simulink model "dc_1"  (Simulink 7.0)
settings: Solver=ode45  StartTime=0.0  StopTime=10.0  MaxStep=1/(2*Fc)  RelTol=1e-3
PreLoadFcn:
  | Fc    =  890e6;
  | Fsym=  20e6;
  | Frame=128;
  | D=8;
  | RRC_Delay;
undefined symbols (not defined in the file): RRC_Delay
libraries: dspbuff3 x4, dsparch4 x4, commfilt2 x2, commsink2 x1, dspstat3 x1, commdigbbndpm3 x1, commrandsrc2 x1
settings Model: Creator=dbenson  LastModifiedBy=dbenson

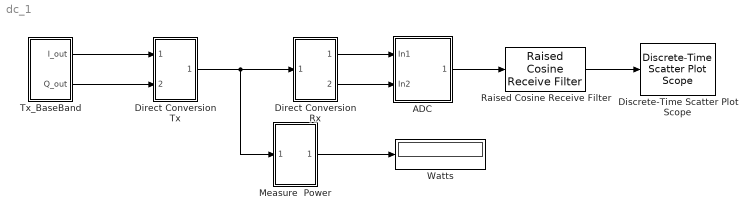
== system dc_1 ==
  ADC : Subsystem
  Direct Conversion Rx : Subsystem
  Direct Conversion Tx : Subsystem
  Discrete-Time Scatter Plot Scope : commsink2/Discrete-Time Scatter Plot Scope  Tag=ScatterPlot  SystemSampleTime=-1  sampPerSymb=1  offsetEye=0  numTraces=40  numNewFrames=10  LineMarkers=.  LineColors=b  fading=on  render=on  AxisGrid=on  xMin=-2.5  xMax=2.5  yMin=-2.5  yMax=2.5  inphaseLabel=In-phase Amplitude  quadratureLabel=Quadrature Amplitude  openScopeAtSimStart=on  FrameNumber=off  FigPos=[786 40 229 225]  figTitle=Scatter Plot  numLinesMax=8  block_type_=scatter
  Measure  Power : Subsystem
  Raised Cosine Receive Filter : commfilt2/Raised Cosine Receive Filter  DialogController=dspDDGCreate  DialogControllerArgs=DataTag1  SystemSampleTime=-1  filtType=Square root  N=8  D=RRC_Delay  R=0.25  sampMode=Frame-based  rateMode=Downsampling  downFactor=D  downOffset=6  checkGain=Normalized  filterGain=1  checkCoeff=off  variableName=rcRxFilt  launchFVT=off  roundingMode=Floor  overflowMode=off
  Tx_BaseBand : Subsystem
  Watts : Display
  wires:
  ADC/1(I/Q out) -> Raised Cosine Receive Filter/1
  Raised Cosine Receive Filter/1 -> Discrete-Time Scatter Plot Scope/1
  Tx_BaseBand/1(I_out) -> Direct Conversion Tx/1(In1)
  Tx_BaseBand/2(Q_out) -> Direct Conversion Tx/2(In2)
  Direct Conversion Rx/1(Out1) -> ADC/1(In1)
  Direct Conversion Rx/2(Out2) -> ADC/2(In2)
  Direct Conversion Tx/1(Out1) -> Direct Conversion Rx/1(In1), Measure  Power/1(In1)
  Measure  Power/1(Out1) -> Watts/1

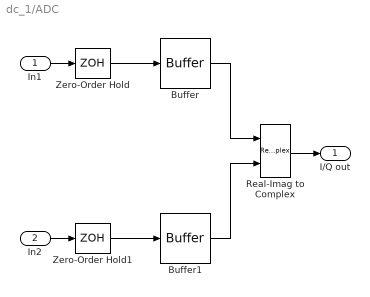
== system dc_1/ADC ==
  In1 : Inport
  In2 : Inport  Port=2
  Buffer : dspbuff3/Buffer  N=Frame  V=0  ic=0
  Buffer1 : dspbuff3/Buffer  N=Frame  V=0  ic=0
  Real-Imag to Complex : RealImagToComplex
  Zero-Order Hold : ZeroOrderHold  SampleTime=1/(D*Fsym)
  Zero-Order Hold1 : ZeroOrderHold  SampleTime=1/(D*Fsym)
  I/Q out : Outport
  wires:
  In1/1 -> Zero-Order Hold/1
  Zero-Order Hold/1 -> Buffer/1
  In2/1 -> Zero-Order Hold1/1
  Zero-Order Hold1/1 -> Buffer1/1
  Buffer/1 -> Real-Imag to Complex/1
  Buffer1/1 -> Real-Imag to Complex/2
  Real-Imag to Complex/1 -> I/Q out/1

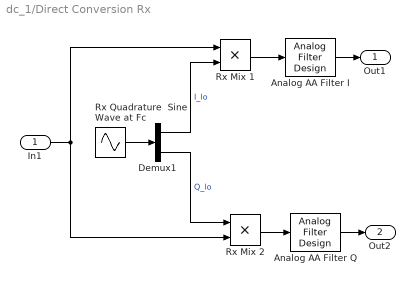
== system dc_1/Direct Conversion Rx ==
  In1 : Inport
  Analog AA Filter I : dsparch4/Analog Filter Design  method=Bessel  filttype=Lowpass  N=5  Wlo=2*pi*2*Fsym  Whi=80  Rp=2  Rs=40
  Analog AA Filter Q : dsparch4/Analog Filter Design  method=Bessel  filttype=Lowpass  N=5  Wlo=2*pi*2*Fsym  Whi=80  Rp=2  Rs=40
  Demux1 : Demux  Outputs=2
  Rx Mix 1 : Product  OutDataType=sfix(16)  OutScaling=2^0  RndMeth=Zero
  Rx Mix 2 : Product  OutDataType=sfix(16)  OutScaling=2^0  RndMeth=Zero
  Rx Quadrature  Sine Wave at Fc : Sin  Frequency=Fc*2*pi  Phase=[-pi/2,0]  SampleTime=0
  Out1 : Outport
  Out2 : Outport  Port=2
  wires:
  In1/1 -> Rx Mix 2/2, Rx Mix 1/1
  Rx Quadrature  Sine Wave at Fc/1 -> Demux1/1
  Demux1/1 -> Rx Mix 1/2  "I_lo"
  Demux1/2 -> Rx Mix 2/1  "Q_lo"
  Rx Mix 1/1 -> Analog AA Filter I/1
  Rx Mix 2/1 -> Analog AA Filter Q/1
  Analog AA Filter I/1 -> Out1/1
  Analog AA Filter Q/1 -> Out2/1

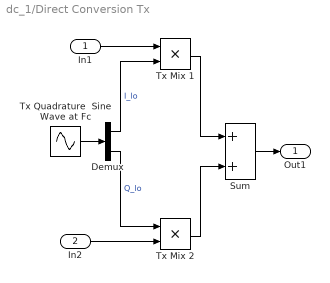
== system dc_1/Direct Conversion Tx ==
  In1 : Inport
  In2 : Inport  Port=2
  Demux : Demux  Outputs=2
  Sum : Sum  OutDataType=sfix(16)  OutScaling=2^0
  Tx Mix 1 : Product  OutDataType=sfix(16)  OutScaling=2^0  RndMeth=Zero
  Tx Mix 2 : Product  OutDataType=sfix(16)  OutScaling=2^0  RndMeth=Zero
  Tx Quadrature  Sine Wave at Fc : Sin  Amplitude=4.1  Frequency=Fc*2*pi  Phase=[-pi/2,0]  SampleTime=0
  Out1 : Outport
  wires:
  Tx Quadrature  Sine Wave at Fc/1 -> Demux/1
  Demux/1 -> Tx Mix 1/2  "I_lo"
  Demux/2 -> Tx Mix 2/1  "Q_lo"
  Tx Mix 1/1 -> Sum/1
  Tx Mix 2/1 -> Sum/2
  In1/1 -> Tx Mix 1/1
  Sum/1 -> Out1/1
  In2/1 -> Tx Mix 2/2

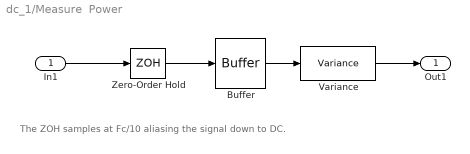
== system dc_1/Measure  Power ==
  note: The ZOH samples at Fc/10
      | aliasing the signal down to DC.
  In1 : Inport
  Buffer : dspbuff3/Buffer  N=Frame*D  V=0  ic=0
  Variance : dspstat3/Variance  DialogController=dspDDGCreate  DialogControllerArgs=DataTag0  run=off  reset_popup=None  roundingMode=Floor  overflowMode=off
  Zero-Order Hold : ZeroOrderHold  SampleTime=10/Fc
  Out1 : Outport
  wires:
  Zero-Order Hold/1 -> Buffer/1
  Buffer/1 -> Variance/1
  In1/1 -> Zero-Order Hold/1
  Variance/1 -> Out1/1

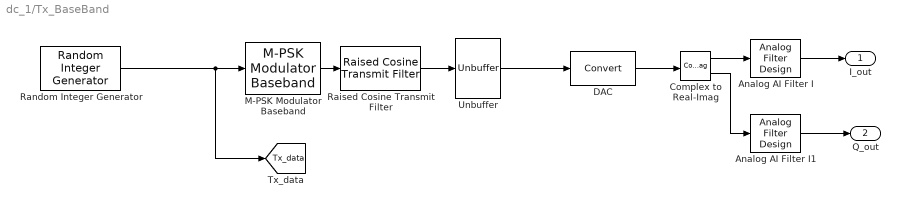
== system dc_1/Tx_BaseBand ==
  Analog AI Filter I : dsparch4/Analog Filter Design  method=Bessel  filttype=Lowpass  N=6  Wlo=2*pi*2*Fsym  Whi=80  Rp=2  Rs=40
  Analog AI Filter I1 : dsparch4/Analog Filter Design  method=Bessel  filttype=Lowpass  N=6  Wlo=2*pi*2*Fsym  Whi=80  Rp=2  Rs=40
  Complex to Real-Imag : ComplexToRealImag
  DAC : DataTypeConversion  OutDataType=sfix(16)  OutScaling=2^0  SampleTime=0
  M-PSK Modulator Baseband : commdigbbndpm3/M-PSK Modulator Baseband  M=4  InType=Integer  Enc=Binary  Mapping=[0:7]  Ph=pi/4  outDtype=double  outWordLen=16  outUDDataType=sfix(16)  outFracLenMode=Best precision  outFracLen=15
  Raised Cosine Transmit Filter : commfilt2/Raised Cosine Transmit Filter  DialogController=dspDDGCreate  DialogControllerArgs=DataTag2  SystemSampleTime=-1  filtType=Square root  D=RRC_Delay  R=0.25  sampMode=Frame-based  N=D  checkGain=Normalized  filterGain=1  checkCoeff=off  variableName=rcTxFilt  launchFVT=off  roundingMode=Floor  overflowMode=off
  Random Integer Generator : commrandsrc2/Random Integer Generator  SystemSampleTime=-1  mul=4  seed=37  Ts=1/Fsym  frameBased=on  sampPerFrame=Frame  orient=off  outDataType=double
  Unbuffer : dspbuff3/Unbuffer  ic=0
  I_out : Outport
  Q_out : Outport  Port=2
  tag scope: Tx_data=global
  wires:
  M-PSK Modulator Baseband/1 -> Raised Cosine Transmit Filter/1
  Raised Cosine Transmit Filter/1 -> Unbuffer/1
  Complex to Real-Imag/1 -> Analog AI Filter I/1
  Complex to Real-Imag/2 -> Analog AI Filter I1/1
  Unbuffer/1 -> DAC/1
  DAC/1 -> Complex to Real-Imag/1
  Random Integer Generator/1 -> M-PSK Modulator Baseband/1, [Tx_data]
  Analog AI Filter I/1 -> I_out/1
  Analog AI Filter I1/1 -> Q_out/1
